simulink model "band_pass_filter_cosim"  (Simulink 7.0)
settings: Solver=VariableStepDiscrete  StartTime=0.0  StopTime=0.35  RelTol=1e-3
undefined symbols (not defined in the file): ieee_nowarn, image, port_label
libraries: aldec_ahdl x6
settings Model: Creator=arekg  LastModifiedBy=arekg
settings OptimizationCC: InlineInvariantSignals=on
settings DebuggingCC: SaveWithParameterizedLinksMsg=none  SignalResolutionControl=TryResolveAllWithWarning  MultiTaskDSMMsg=warning  MultiTaskCondExecSysMsg=none
settings RTWCC: IncludeERTFirstTime=on
settings GRTTargetCC: TargetFcnLib=ansi_tfl_tmw.mat

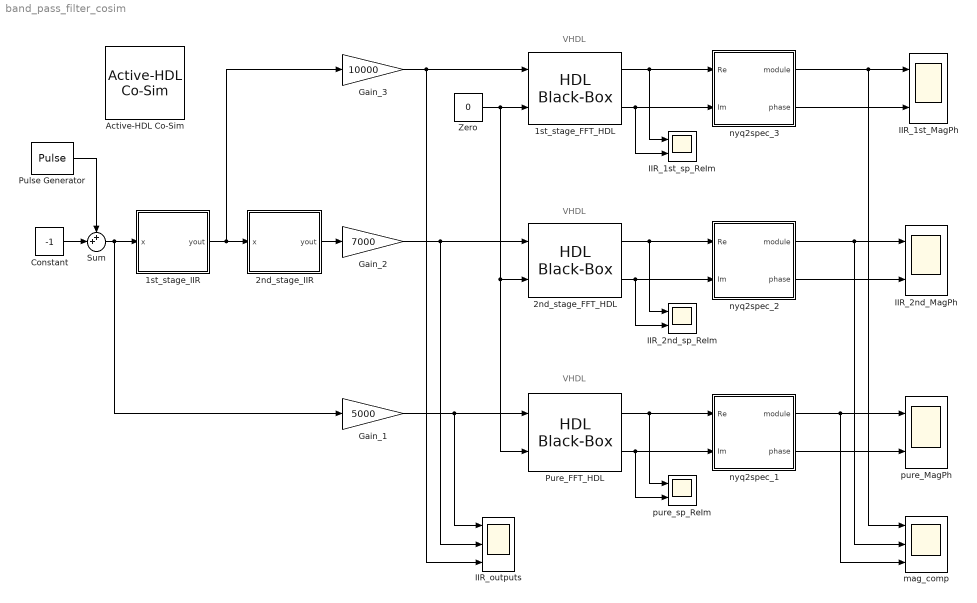
== system band_pass_filter_cosim ==
  note: VHDL
  note: VHDL
  note: VHDL
  1st_stage_FFT_HDL : aldec_ahdl/HDL Black-Box  module_m=top_fft  ports_cfg={ce,4,1,2,0,1,8,0,0,1,0,0}{clk,3,1,2,0,1,8,0,0,1,0,0}{inv,5,1,2,0,1,8,0,0,1,0,0}{rst,5,1,2,0,1,8,0,0,1,0,0}{start,5,1,2,0,1,8,0,0,1,0,0}{Iin,0,-1,2,0,1,0,0,0,0,0,0}{Qin,0,-1,2,0,1,0,0,0,0,0,0}{Iout,1,-1,2,0,ce,0,0,0,0,0,0}{Qout,1,-1,2,0,ce,0,0,0,0,0,0}  params={WIDTH,16,NATURAL}{POINT,1024,NATURAL}{STAGE,5,NATURAL}  clocks={1,2,0,0.5000,0}  ces={0,1,4,0,1}  stims={3,1 0ns 0 320us}{4,0 0ns 1 380us 0 480us}{2,0}  hdl_src=c:\My_Designs\Samples_83\simulink_band_pass_filter\fft\compile\top_fft.vhd;c:\My_Designs\Samples_83\simulink_band_pass_filter\fft\src\cfft\address.vhd;c:\My_Designs\Samples_83\simulink_band_pass_filter\fft\src\cfft\blockdram.vhd;c:\My_Designs\Samples_83\simulink_band_pass_filter\fft\src\cfft\div4limit.vhd;c:\My_Designs\Samples_83\simulink_band_pass_filter\fft\src\cfft\cfft4.vhd;c:\My_Designs\Samples_83\simulink_band_pass_filter\fft\src\cfft\rofactor.vhd;c:\My_Designs\Samples_83\simulink_band_pass_filter\fft\src\cfft\p2r_cordic.vhd;c:\My_Designs\Samples_83\simulink_band_pass_filter\fft\src\cfft\sc_corproc.vhd;c:\My_Designs\Samples_83\simulink_band_pass_filter\fft\src\cfft\mulfactor.vhd;c:\My_Designs\Samples_83\simulink_band_pass_filter\fft\src\cfft\cfft.vhd;c:\My_Designs\Samples_83\simulink_band_pass_filter\fft\src\ram\ram.vhd;c:\My_Designs\Samples_83\simulink_band_pass_filter\fft\compile\control.vhd  block_mask=image(imread('HDLBlackBox.jpg'),'center'); disp('top_fft');port_label('input', 1, 'Iin');port_label('input', 2, 'Qin');port_label('output', 1, 'Iout');port_label('output', 2, 'Qout');  config=[2,2]  inp=[2, 0, abs(16-1 - 0) + 1, 0, 0, 0, 2, 0, abs(16-1 - 0) + 1, 0, 0, 0, 2]  out=[2, 0, abs(16+1 - 0) + 1, 0, 0, 0, 2, 0, abs(16+1 - 0) + 1, 0, 0, 0, 2]  sampling=[0,1,1,4*2,4*2]  active_page={5}{80,0,35,1,65,2,70,3,70,4,60,5,60,6,50,7,35,8,35,9,119,10}{103,0,55,1,70,2,75,3,75,4,45,5,45,6,45,7,165,8,0,0,0,0}{165,0,130,1,190,2,190,3,0,0,0,0,0,0,0,0,0,0,0,0,0,0}{81,0,60,1,60,2,70,3,60,4,0,0,0,0,0,0,0,0,0,0,0,0}{83,0,70,1,80,2,50,3,50,4,0,0,0,0,0,0,0,0,0,0,0,0}{125,0,330,1,220,2,0,0,0,0,0,0,0,0,0,0,0,0,0,0,0,0}{95,0,95,1,70,2,50,3,80,4,35,5,35,6,65,7,150,8,0,0,0,0}{735,436}  param_val={16,-1,1024,-1,5,-1}  clk_val=[2,0,0.5000]  ce_val=[4,0]  blk_ver=9.1.RTM  blk_conf=0  user_conv=0
  1st_stage_IIR : Subsystem
  2nd_stage_FFT_HDL : aldec_ahdl/HDL Black-Box  module_m=top_fft  ports_cfg={ce,4,1,2,0,1,8,0,0,1,0,0}{clk,3,1,2,0,1,8,0,0,1,0,0}{inv,5,1,2,0,1,8,0,0,1,0,0}{rst,5,1,2,0,1,8,0,0,1,0,0}{start,5,1,2,0,1,8,0,0,1,0,0}{Iin,0,-1,2,0,1,0,0,0,0,0,0}{Qin,0,-1,2,0,1,0,0,0,0,0,0}{Iout,1,-1,2,0,ce,0,0,0,0,0,0}{Qout,1,-1,2,0,ce,0,0,0,0,0,0}  params={WIDTH,16,NATURAL}{POINT,1024,NATURAL}{STAGE,5,NATURAL}  clocks={1,2,0,0.5000,0}  ces={0,1,4,0,1}  stims={3,1 0ns 0 320us}{4,0 0ns 1 380us 0 480us}{2,0}  hdl_src=c:\My_Designs\Samples_83\simulink_band_pass_filter\fft\compile\top_fft.vhd;c:\My_Designs\Samples_83\simulink_band_pass_filter\fft\src\cfft\address.vhd;c:\My_Designs\Samples_83\simulink_band_pass_filter\fft\src\cfft\blockdram.vhd;c:\My_Designs\Samples_83\simulink_band_pass_filter\fft\src\cfft\div4limit.vhd;c:\My_Designs\Samples_83\simulink_band_pass_filter\fft\src\cfft\cfft4.vhd;c:\My_Designs\Samples_83\simulink_band_pass_filter\fft\src\cfft\rofactor.vhd;c:\My_Designs\Samples_83\simulink_band_pass_filter\fft\src\cfft\p2r_cordic.vhd;c:\My_Designs\Samples_83\simulink_band_pass_filter\fft\src\cfft\sc_corproc.vhd;c:\My_Designs\Samples_83\simulink_band_pass_filter\fft\src\cfft\mulfactor.vhd;c:\My_Designs\Samples_83\simulink_band_pass_filter\fft\src\cfft\cfft.vhd;c:\My_Designs\Samples_83\simulink_band_pass_filter\fft\src\ram\ram.vhd;c:\My_Designs\Samples_83\simulink_band_pass_filter\fft\compile\control.vhd  block_mask=image(imread('HDLBlackBox.jpg'),'center'); disp('top_fft');port_label('input', 1, 'Iin');port_label('input', 2, 'Qin');port_label('output', 1, 'Iout');port_label('output', 2, 'Qout');  config=[2,2]  inp=[2, 0, abs(16-1 - 0) + 1, 0, 0, 0, 2, 0, abs(16-1 - 0) + 1, 0, 0, 0, 2]  out=[2, 0, abs(16+1 - 0) + 1, 0, 0, 0, 2, 0, abs(16+1 - 0) + 1, 0, 0, 0, 2]  sampling=[0,1,1,4*2,4*2]  active_page={0}{80,0,35,1,65,2,70,3,70,4,60,5,60,6,50,7,35,8,35,9,119,10}{103,0,55,1,70,2,75,3,75,4,45,5,45,6,45,7,165,8,0,0,0,0}{165,0,130,1,190,2,190,3,0,0,0,0,0,0,0,0,0,0,0,0,0,0}{81,0,60,1,60,2,70,3,60,4,0,0,0,0,0,0,0,0,0,0,0,0}{83,0,70,1,80,2,50,3,50,4,0,0,0,0,0,0,0,0,0,0,0,0}{125,0,330,1,220,2,0,0,0,0,0,0,0,0,0,0,0,0,0,0,0,0}{95,0,95,1,70,2,50,3,80,4,35,5,35,6,65,7,150,8,0,0,0,0}{735,436}  param_val={16,-1,1024,-1,5,-1}  clk_val=[2,0,0.5000]  ce_val=[4,0]  blk_ver=9.1.RTM  blk_conf=0  user_conv=0
  2nd_stage_IIR : Subsystem
  Active-HDL Co-Sim : aldec_ahdl/Active-HDL Co-Sim  Tag=Active-HDL_Co-Sim_close  hdl_period=176  hdl_tscale=kHz  sys_period=[176, 0]  sys_tscale=As In Simulator  vsim_cmd=-ieee_nowarn  wav_fn=band_pass_filter_cosim  wav_settings=[0,0,0,0,0,0,0,0]  dbg=off  auto_start=off  gen_tb=[0,0]  batch_sim=off  tb_fn=mlab_post_tb.log  metavalue_map=[0,0]  sim_resolution=[1,0,0]  active_page=0  aws_en=off  ahdl_en=off  blk_ver=9.1.RTM  macro_en=[1,0,1]  macro_path=prepare_project.do  mfun_text=check_mfiles
  Constant : Constant  Value=-1  OutDataType=sfix(16)  OutScaling=2^0
  Gain_1 : Gain  Gain=5000  ParameterDataType=sfix(16)  ParameterScaling=2^0  OutDataType=sfix(16)  OutScaling=2^0
  Gain_2 : Gain  Gain=7000  ParameterDataType=sfix(16)  ParameterScaling=2^0  OutDataType=sfix(16)  OutScaling=2^0
  Gain_3 : Gain  Gain=10000  ParameterDataType=sfix(16)  ParameterScaling=2^0  OutDataType=sfix(16)  OutScaling=2^0
  IIR_1st_MagPh : Scope  NumInputPorts=2
      settings: TimeRange=0.35  YMin=0~-4  YMax=80000~4  SaveName=ScopeData8
  IIR_1st_sp_ReIm : Scope  NumInputPorts=2
      settings: TimeRange=0.35  YMin=-80000~-15000  YMax=40000~15000  SaveName=ScopeData9
  IIR_2nd_MagPh : Scope  NumInputPorts=2
      settings: TimeRange=0.35  YMin=0~-4  YMax=90000~4
  IIR_2nd_sp_ReIm : Scope  NumInputPorts=2
      settings: TimeRange=0.35  YMin=-40000~-25000  YMax=80000~25000
  IIR_outputs : Scope  NumInputPorts=3
      settings: TimeRange=0.004173519736842107  YMin=-1~-1~-1  YMax=1~1~1  SaveName=ScopeData6
  Pulse Generator : DiscretePulseGenerator  PulseType=Time based  Amplitude=2  Period=1/1000  PulseWidth=50  VectorParams1D=off
  Pure_FFT_HDL : aldec_ahdl/HDL Black-Box  module_m=top_fft  ports_cfg={ce,4,1,2,0,1,8,0,0,1,0,0}{clk,3,1,2,0,1,8,0,0,1,0,0}{inv,5,1,2,0,1,8,0,0,1,0,0}{rst,5,1,2,0,1,8,0,0,1,0,0}{start,5,1,2,0,1,8,0,0,1,0,0}{Iin,0,-1,2,0,1,0,0,0,0,0,0}{Qin,0,-1,2,0,1,0,0,0,0,0,0}{Iout,1,-1,2,0,ce,0,0,0,0,0,0}{Qout,1,-1,2,0,ce,0,0,0,0,0,0}  params={WIDTH,16,NATURAL}{POINT,1024,NATURAL}{STAGE,5,NATURAL}  clocks={1,2,0,0.5000,0}  ces={0,1,4,0,1}  stims={3,1 0ns 0 320us}{4,0 0ns 1 380us 0 480us}{2,0}  hdl_src=c:\My_Designs\Samples_83\simulink_band_pass_filter\fft\compile\top_fft.vhd;c:\My_Designs\Samples_83\simulink_band_pass_filter\fft\src\cfft\address.vhd;c:\My_Designs\Samples_83\simulink_band_pass_filter\fft\src\cfft\blockdram.vhd;c:\My_Designs\Samples_83\simulink_band_pass_filter\fft\src\cfft\div4limit.vhd;c:\My_Designs\Samples_83\simulink_band_pass_filter\fft\src\cfft\cfft4.vhd;c:\My_Designs\Samples_83\simulink_band_pass_filter\fft\src\cfft\rofactor.vhd;c:\My_Designs\Samples_83\simulink_band_pass_filter\fft\src\cfft\p2r_cordic.vhd;c:\My_Designs\Samples_83\simulink_band_pass_filter\fft\src\cfft\sc_corproc.vhd;c:\My_Designs\Samples_83\simulink_band_pass_filter\fft\src\cfft\mulfactor.vhd;c:\My_Designs\Samples_83\simulink_band_pass_filter\fft\src\cfft\cfft.vhd;c:\My_Designs\Samples_83\simulink_band_pass_filter\fft\src\ram\ram.vhd;c:\My_Designs\Samples_83\simulink_band_pass_filter\fft\compile\control.vhd  block_mask=image(imread('HDLBlackBox.jpg'),'center'); disp('top_fft');port_label('input', 1, 'Iin');port_label('input', 2, 'Qin');port_label('output', 1, 'Iout');port_label('output', 2, 'Qout');  config=[2,2]  inp=[2, 0, abs(16-1 - 0) + 1, 0, 0, 0, 2, 0, abs(16-1 - 0) + 1, 0, 0, 0, 2]  out=[2, 0, abs(16+1 - 0) + 1, 0, 0, 0, 2, 0, abs(16+1 - 0) + 1, 0, 0, 0, 2]  sampling=[0,1,1,4*2,4*2]  active_page={0}{80,0,35,1,65,2,70,3,70,4,60,5,60,6,50,7,35,8,35,9,119,10}{103,0,55,1,70,2,75,3,75,4,45,5,45,6,45,7,165,8,0,0,0,0}{165,0,130,1,190,2,190,3,0,0,0,0,0,0,0,0,0,0,0,0,0,0}{81,0,60,1,60,2,70,3,60,4,0,0,0,0,0,0,0,0,0,0,0,0}{83,0,70,1,80,2,50,3,50,4,0,0,0,0,0,0,0,0,0,0,0,0}{125,0,330,1,220,2,0,0,0,0,0,0,0,0,0,0,0,0,0,0,0,0}{95,0,95,1,70,2,50,3,80,4,35,5,35,6,65,7,150,8,0,0,0,0}{735,436}  param_val={16,-1,1024,-1,5,-1}  clk_val=[2,0,0.5000]  ce_val=[4,0]  blk_ver=9.1.RTM  blk_conf=0  user_conv=0
  Sum : Sum  Inputs=++|  OutDataType=sfix(16)  OutScaling=2^0
  Zero : Constant  Value=0  OutDataType=sfix(16)  OutScaling=2^0
  mag_comp : Scope  NumInputPorts=3
      settings: TimeRange=0.35  YMin=0~0~0  YMax=40000~20000~80000  SaveName=ScopeData5
  nyq2spec_1 : Subsystem
  nyq2spec_2 : Subsystem
  nyq2spec_3 : Subsystem
  pure_MagPh : Scope  NumInputPorts=2
      settings: TimeRange=0.35  YMin=0~-4  YMax=70000~4  SaveName=ScopeData3
  pure_sp_ReIm : Scope  NumInputPorts=2
      settings: TimeRange=0.35  YMin=-60000~-25  YMax=80000~20  SaveName=ScopeData4
  wires:
  1st_stage_IIR/1(yout) -> 2nd_stage_IIR/1(x), Gain_3/1
  Sum/1 -> 1st_stage_IIR/1(x), Gain_1/1
  2nd_stage_FFT_HDL/1 -> IIR_2nd_sp_ReIm/1, nyq2spec_2/1(Re)
  2nd_stage_FFT_HDL/2 -> IIR_2nd_sp_ReIm/2, nyq2spec_2/2(Im)
  nyq2spec_2/1(module) -> IIR_2nd_MagPh/1, mag_comp/2
  nyq2spec_2/2(phase) -> IIR_2nd_MagPh/2
  Pure_FFT_HDL/1 -> pure_sp_ReIm/1, nyq2spec_1/1(Re)
  Pure_FFT_HDL/2 -> pure_sp_ReIm/2, nyq2spec_1/2(Im)
  nyq2spec_1/1(module) -> pure_MagPh/1, mag_comp/3
  nyq2spec_1/2(phase) -> pure_MagPh/2
  Gain_2/1 -> 2nd_stage_FFT_HDL/1, IIR_outputs/2
  Gain_1/1 -> Pure_FFT_HDL/1, IIR_outputs/1
  2nd_stage_IIR/1(yout) -> Gain_2/1
  Zero/1 -> Pure_FFT_HDL/2, 2nd_stage_FFT_HDL/2, 1st_stage_FFT_HDL/2
  1st_stage_FFT_HDL/1 -> IIR_1st_sp_ReIm/1, nyq2spec_3/1(Re)
  1st_stage_FFT_HDL/2 -> IIR_1st_sp_ReIm/2, nyq2spec_3/2(Im)
  nyq2spec_3/1(module) -> IIR_1st_MagPh/1, mag_comp/1
  nyq2spec_3/2(phase) -> IIR_1st_MagPh/2
  Gain_3/1 -> 1st_stage_FFT_HDL/1, IIR_outputs/3
  Constant/1 -> Sum/2
  Pulse Generator/1 -> Sum/1

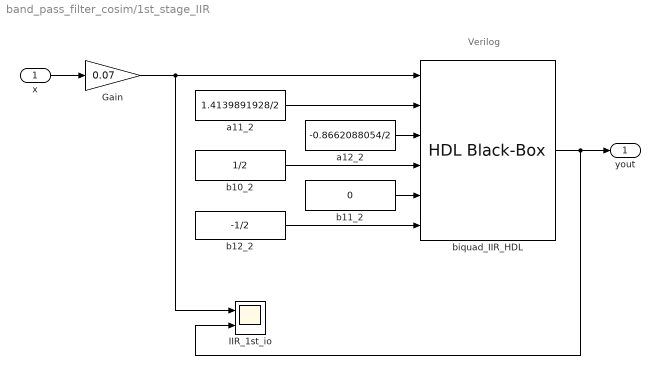
== system band_pass_filter_cosim/1st_stage_IIR ==
  note: Verilog
  x : Inport  OutDataType=sfix(16)  OutScaling=2^0
  Gain : Gain  Gain=0.07  ParameterDataType=sfix(16)  ParameterScaling=2^0  OutDataType=sfix(16)  OutScaling=2^0  SaturateOnIntegerOverflow=on
  IIR_1st_io : Scope  NumInputPorts=2
      settings: TimeRange=0.006433823529411766  YMin=-0.08~-1  YMax=0.08~1  SaveName=ScopeData2
  a11_2 : Constant  Value=1.4139891928/2  OutDataType=sfix(16)  OutScaling=2^0
  a12_2 : Constant  Value=-0.8662088054/2  OutDataType=sfix(16)  OutScaling=2^0
  b10_2 : Constant  Value=1/2  OutDataType=sfix(16)  OutScaling=2^0
  b11_2 : Constant  Value=0  OutDataType=sfix(16)  OutScaling=2^0
  b12_2 : Constant  Value=-1/2  OutDataType=sfix(16)  OutScaling=2^0
  biquad_IIR_HDL : aldec_ahdl/HDL Black-Box  module_m=biquad  ports_cfg={clk,3,1,2,0,1,8,0,0,1,0,0}{nreset,5,1,2,0,1,8,0,0,1,0,0}{x,0,16,2,15,1,0,0,0,0,0,0}{ce,4,1,2,0,1,8,0,0,1,0,0}{valid,5,1,2,0,1,8,0,0,1,0,0}{a11,0,8,2,7,1,0,0,0,0,0,0}{a12,0,8,2,7,1,0,0,0,0,0,0}{b10,0,8,2,7,1,0,0,0,0,0,0}{b11,0,8,2,7,1,0,0,0,0,0,0}{b12,0,8,2,7,1,0,0,0,0,0,0}{yout,1,16,2,15,ce,0,0,0,0,0,0}  params={DATAWIDTH,16,}{COEFWIDTH,8,}{ACCUM,2,}  clocks={0,2,0,0.5000,0}  ces={3,0,2,0,1}  stims={1,0 0us 1 45us}{4,0 0us 1 45us}  hdl_src=c:\My_Designs\Samples_83\simulink_band_pass_filter\biquad_iir\src\multa.v;c:\My_Designs\Samples_83\simulink_band_pass_filter\biquad_iir\src\multb.v;c:\My_Designs\Samples_83\simulink_band_pass_filter\biquad_iir\src\biquad.v  block_mask=image(imread('HDLBlackBox.jpg'),'center'); disp('biquad');port_label('input', 1, 'x');port_label('input', 2, 'a11');port_label('input', 3, 'a12');port_label('input', 4, 'b10');port_label('input', 5, 'b11');port_label('input', 6, 'b12');port_label('output', 1, 'yout');  config=[6,1]  inp=[6, 0, 16, 15, 0, 0, 2, 0, 8, 7, 0, 0, 2, 0, 8, 7, 0, 0, 2, 0, 8, 7, 0, 0, 2, 0, 8, 7, 0, 0, 2, 0, 8, 7, 0, 0, 2]  out=[1, 0, 16, 15, 0, 0, 2]  sampling=[0,1,1,1,1,1,1,2*2]  active_page={0}{80,0,35,1,65,2,70,3,70,4,60,5,60,6,50,7,35,8,35,9,119,10}{103,0,55,1,70,2,75,3,75,4,45,5,45,6,45,7,165,8,0,0,0,0}{165,0,130,1,190,2,190,3,0,0,0,0,0,0,0,0,0,0,0,0,0,0}{81,0,60,1,60,2,70,3,60,4,0,0,0,0,0,0,0,0,0,0,0,0}{83,0,70,1,80,2,50,3,50,4,0,0,0,0,0,0,0,0,0,0,0,0}{125,0,330,1,220,2,0,0,0,0,0,0,0,0,0,0,0,0,0,0,0,0}{95,0,95,1,70,2,50,3,80,4,35,5,35,6,65,7,150,8,0,0,0,0}{735,436}  param_val={16,-1,8,-1,2,-1}  clk_val=[2,0,0.5000]  ce_val=[2,0]  blk_ver=9.1.RTM  blk_conf=0  user_conv=0
  yout : Outport  OutDataType=sfix(16)  OutScaling=2^0
  wires:
  x/1 -> Gain/1
  Gain/1 -> IIR_1st_io/1, biquad_IIR_HDL/1
  b12_2/1 -> biquad_IIR_HDL/6
  b10_2/1 -> biquad_IIR_HDL/4
  a12_2/1 -> biquad_IIR_HDL/3
  a11_2/1 -> biquad_IIR_HDL/2
  b11_2/1 -> biquad_IIR_HDL/5
  biquad_IIR_HDL/1 -> yout/1, IIR_1st_io/2

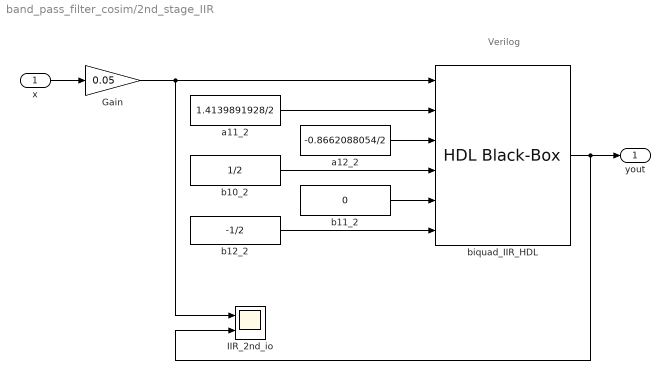
== system band_pass_filter_cosim/2nd_stage_IIR ==
  note: Verilog
  x : Inport  OutDataType=sfix(16)  OutScaling=2^0
  Gain : Gain  Gain=0.05  ParameterDataType=sfix(16)  ParameterScaling=2^0  OutDataType=sfix(16)  OutScaling=2^0  SaturateOnIntegerOverflow=on
  IIR_2nd_io : Scope  NumInputPorts=2
      settings: TimeRange=0.006433823529411766  YMin=-0.08~-1  YMax=0.08~1  SaveName=ScopeData7
  a11_2 : Constant  Value=1.4139891928/2  OutDataType=sfix(16)  OutScaling=2^0
  a12_2 : Constant  Value=-0.8662088054/2  OutDataType=sfix(16)  OutScaling=2^0
  b10_2 : Constant  Value=1/2  OutDataType=sfix(16)  OutScaling=2^0
  b11_2 : Constant  Value=0  OutDataType=sfix(16)  OutScaling=2^0
  b12_2 : Constant  Value=-1/2  OutDataType=sfix(16)  OutScaling=2^0
  biquad_IIR_HDL : aldec_ahdl/HDL Black-Box  module_m=biquad  ports_cfg={clk,3,1,2,0,1,8,0,0,1,0,0}{nreset,5,1,2,0,1,8,0,0,1,0,0}{x,0,16,2,15,1,0,0,0,0,0,0}{ce,4,1,2,0,1,8,0,0,1,0,0}{valid,5,1,2,0,1,8,0,0,1,0,0}{a11,0,8,2,7,1,0,0,0,0,0,0}{a12,0,8,2,7,1,0,0,0,0,0,0}{b10,0,8,2,7,1,0,0,0,0,0,0}{b11,0,8,2,7,1,0,0,0,0,0,0}{b12,0,8,2,7,1,0,0,0,0,0,0}{yout,1,16,2,15,ce,0,0,0,0,0,0}  params={DATAWIDTH,16,}{COEFWIDTH,8,}{ACCUM,2,}  clocks={0,2,0,0.5000,0}  ces={3,0,2,0,1}  stims={1,0 0us 1 45us}{4,0 0us 1 45us}  hdl_src=c:\My_Designs\Samples_83\simulink_band_pass_filter\biquad_iir\src\multa.v;c:\My_Designs\Samples_83\simulink_band_pass_filter\biquad_iir\src\multb.v;c:\My_Designs\Samples_83\simulink_band_pass_filter\biquad_iir\src\biquad.v  block_mask=image(imread('HDLBlackBox.jpg'),'center'); disp('biquad');port_label('input', 1, 'x');port_label('input', 2, 'a11');port_label('input', 3, 'a12');port_label('input', 4, 'b10');port_label('input', 5, 'b11');port_label('input', 6, 'b12');port_label('output', 1, 'yout');  config=[6,1]  inp=[6, 0, 16, 15, 0, 0, 2, 0, 8, 7, 0, 0, 2, 0, 8, 7, 0, 0, 2, 0, 8, 7, 0, 0, 2, 0, 8, 7, 0, 0, 2, 0, 8, 7, 0, 0, 2]  out=[1, 0, 16, 15, 0, 0, 2]  sampling=[0,1,1,1,1,1,1,2*2]  active_page={0}{80,0,35,1,65,2,70,3,70,4,60,5,60,6,50,7,35,8,35,9,119,10}{103,0,55,1,70,2,75,3,75,4,45,5,45,6,45,7,165,8,0,0,0,0}{165,0,130,1,190,2,190,3,0,0,0,0,0,0,0,0,0,0,0,0,0,0}{81,0,60,1,60,2,70,3,60,4,0,0,0,0,0,0,0,0,0,0,0,0}{83,0,70,1,80,2,50,3,50,4,0,0,0,0,0,0,0,0,0,0,0,0}{125,0,330,1,220,2,0,0,0,0,0,0,0,0,0,0,0,0,0,0,0,0}{95,0,95,1,70,2,50,3,80,4,35,5,35,6,65,7,150,8,0,0,0,0}{735,436}  param_val={16,-1,8,-1,2,-1}  clk_val=[2,0,0.5000]  ce_val=[2,0]  blk_ver=9.1.RTM  blk_conf=0  user_conv=0
  yout : Outport  OutDataType=sfix(16)  OutScaling=2^0
  wires:
  x/1 -> Gain/1
  Gain/1 -> IIR_2nd_io/1, biquad_IIR_HDL/1
  b12_2/1 -> biquad_IIR_HDL/6
  b10_2/1 -> biquad_IIR_HDL/4
  a12_2/1 -> biquad_IIR_HDL/3
  a11_2/1 -> biquad_IIR_HDL/2
  b11_2/1 -> biquad_IIR_HDL/5
  biquad_IIR_HDL/1 -> yout/1, IIR_2nd_io/2

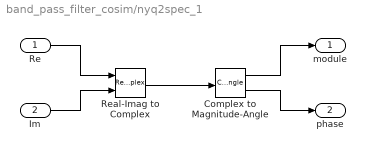
== system band_pass_filter_cosim/nyq2spec_1 ==
  Re : Inport  OutDataType=sfix(16)  OutScaling=2^0
  Im : Inport  Port=2  OutDataType=sfix(16)  OutScaling=2^0
  Complex to Magnitude-Angle : ComplexToMagnitudeAngle
  Real-Imag to Complex : RealImagToComplex
  module : Outport  OutDataType=sfix(16)  OutScaling=2^0
  phase : Outport  Port=2  OutDataType=sfix(16)  OutScaling=2^0
  wires:
  Re/1 -> Real-Imag to Complex/1
  Real-Imag to Complex/1 -> Complex to Magnitude-Angle/1
  Complex to Magnitude-Angle/1 -> module/1
  Im/1 -> Real-Imag to Complex/2
  Complex to Magnitude-Angle/2 -> phase/1

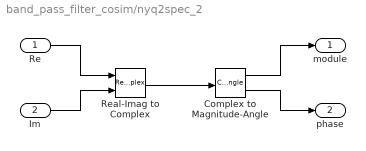
== system band_pass_filter_cosim/nyq2spec_2 ==
  Re : Inport  OutDataType=sfix(16)  OutScaling=2^0
  Im : Inport  Port=2  OutDataType=sfix(16)  OutScaling=2^0
  Complex to Magnitude-Angle : ComplexToMagnitudeAngle
  Real-Imag to Complex : RealImagToComplex
  module : Outport  OutDataType=sfix(16)  OutScaling=2^0
  phase : Outport  Port=2  OutDataType=sfix(16)  OutScaling=2^0
  wires:
  Re/1 -> Real-Imag to Complex/1
  Real-Imag to Complex/1 -> Complex to Magnitude-Angle/1
  Complex to Magnitude-Angle/1 -> module/1
  Im/1 -> Real-Imag to Complex/2
  Complex to Magnitude-Angle/2 -> phase/1

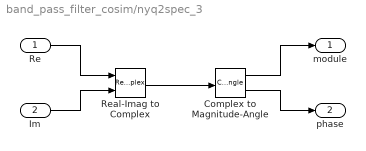
== system band_pass_filter_cosim/nyq2spec_3 ==
  Re : Inport  OutDataType=sfix(16)  OutScaling=2^0
  Im : Inport  Port=2  OutDataType=sfix(16)  OutScaling=2^0
  Complex to Magnitude-Angle : ComplexToMagnitudeAngle
  Real-Imag to Complex : RealImagToComplex
  module : Outport  OutDataType=sfix(16)  OutScaling=2^0
  phase : Outport  Port=2  OutDataType=sfix(16)  OutScaling=2^0
  wires:
  Re/1 -> Real-Imag to Complex/1
  Real-Imag to Complex/1 -> Complex to Magnitude-Angle/1
  Complex to Magnitude-Angle/1 -> module/1
  Im/1 -> Real-Imag to Complex/2
  Complex to Magnitude-Angle/2 -> phase/1
